simulink model "Core_Model_Cal"  (R2023a)
settings: Solver=FixedStepAuto  StartTime=0  StopTime=Z  FixedStep=1/24  RelTol=1e-3
values from neighbouring files (symbols this model uses):
  c_eh = 0.85    [Model_Parameters.m]
  cc_e = -0.85    [Model_Parameters.m]
  R_H2 = 0.05    [Model_Parameters.m]
  R_lh = 0.025    [Model_Parameters.m]
  R_ng = 0.025    [Model_Parameters.m]
libraries: fl_lib x62, nesl_utility x46, ee_lib x22
settings Model: Creator=pienv  LastModifiedBy=pienv

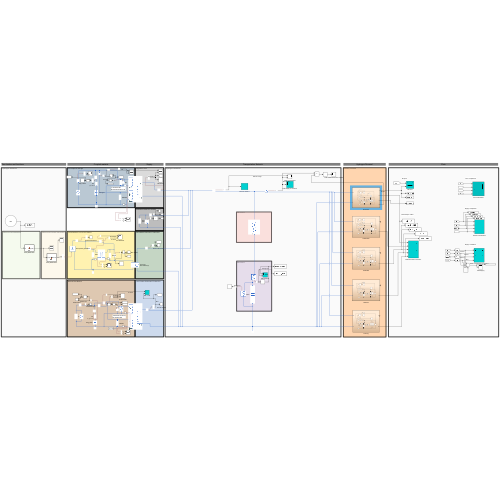
[thumbnail: Simulink's stored preview of the top-level diagram]
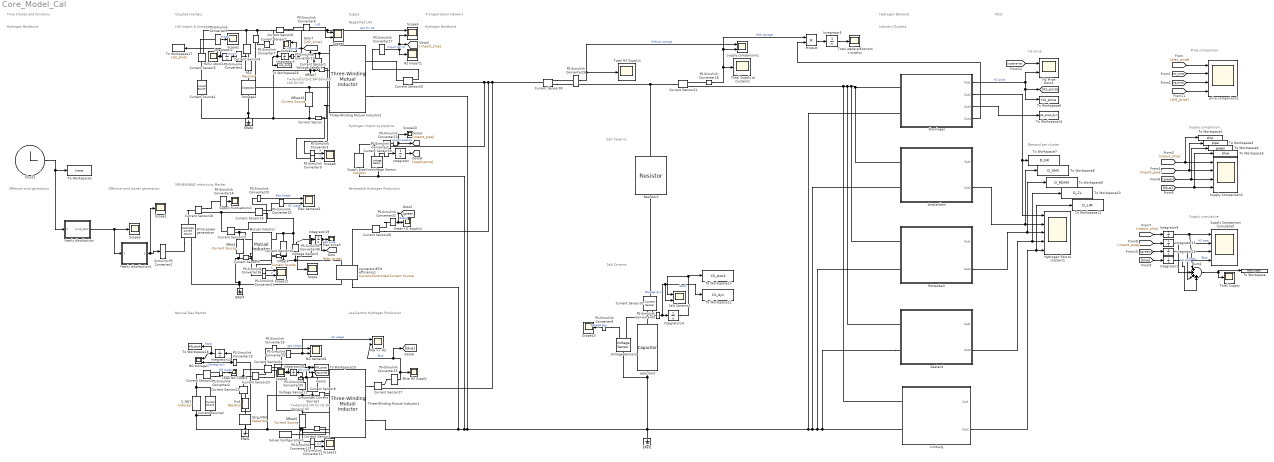
== system Core_Model_Cal ==
  note: Price comparison
  note: Hydrogen Backbone
  note: Supply comparison
  note: Demand per cluster
  note: H2 price
  note: Supply cumulative
  note: Hydrogen Import by pipeline
  note: Renewable Hydrogen Production
  note: Offshore wind generation
  note: Plots
  note: Coupled markets
  note: Natural Gas Market
  note: LH2 Import & storage
  note: Transportation Network
  note: Industry Clusters
  note: Hydrogen Demand
  note: Supply
  note: Offshore wind power generation
  note: Time tracker and functions
  note: T=demand NG for H2
      | B= demand NG
  note: Low-Carbon Hydrogen Production
  note: Salt Caverns
  note: Regasified LH2
  note: Salt Caverns
  note: T=demand LH2
      | B= demand LH2 for H2
  note: Hydrogen Backbone
  note: (RENEWABLE) electricity Market
  Amsterdam : Subsystem
  Blue H2 Supply : Scope
  Clock1 : Clock
      settings: Decimation=24
  Current Sensor{,1..10,17..25,27..28,30..31} (24 alike) : fl_lib/Electrical/Electrical Sensors/Current Sensor
  Current Source1 : ee_lib/Sources/Current Source  dc_current=I_LH2 A  ac_current=0 A  ac_shift=0 rad  ac_frequency=60 Hz  noise_mode=ee.enum.sources.noise.Disabled  PSD=0 A^2/Hz  sample_time=1e-3 s  repeatability=ee.enum.sources.repeatability.NotRepeatable  user_seed=0  auto_seed=3890346746  i_specify=off  i_priority=None  i=0 A  i_nominal_specify=off  i_nominal_unit=A  i_nominal_value=1  v_specify=off  v_priority=None  v=0 V  v_nominal_specify=off  v_nominal_unit=V  v_nominal_value=1
  Current Source2 : ee_lib/Sources/Current Source  dc_current=v_sng A  ac_current=0 A  ac_shift=0 rad  ac_frequency=60 Hz  noise_mode=ee.enum.sources.noise.Disabled  PSD=0 A^2/Hz  sample_time=1e-3 s  repeatability=ee.enum.sources.repeatability.NotRepeatable  user_seed=0  auto_seed=545404223  i_specify=off  i_priority=None  i=0 A  i_nominal_specify=off  i_nominal_unit=A  i_nominal_value=1  v_specify=off  v_priority=None  v=0 V  v_nominal_specify=off  v_nominal_unit=V  v_nominal_value=1
  ERef{1..4} (4 alike) : fl_lib/Electrical/Electrical Elements/Electrical Reference
  Elec demand1 : Scope  NumInputPorts=2
  Elec price3 : Scope
  Green H2 supply1 : Scope
  Groningen : Subsystem
  H2 Import1 : Scope
  H2 Price : Scope  NumInputPorts=2
  H2(L) stock1 : Scope
  Hydrogen flow to clusters1 : Scope  NumInputPorts=5
  Integrator{,1..3,5,9,12,14..16,19..20} (12 alike) : Integrator
  Limburg : Subsystem
  Mutual Inductor : fl_lib/Electrical/Electrical Elements/Mutual Inductor  L1=L_eh H  L2=L_e H  k=cc_e  i1_specify=off  i1_priority=High  i1=0 A  i1_nominal_specify=off  i1_nominal_unit=A  i1_nominal_value=1  i2_specify=off  i2_priority=High  i2=0 A  i2_nominal_specify=off  i2_nominal_unit=A  i2_nominal_value=1  v1_specify=off  v1_priority=None  v1=0 V  v1_nominal_specify=off  v1_nominal_unit=V  v1_nominal_value=1  v2_specify=off  v2_priority=None  v2=0 V  v2_nominal_specify=off  v2_nominal_unit=V  v2_nominal_value=1
      settings: InternalSimscapePortConfiguration="{\"Bottom\":[],\"Left\":[{\"id\":\"p1\",\"label\":\"1+\",\"type\":\"foundation.electrical.electrical\"},{\"id\":\"n1\",\"label\":\"1-\",\"type\":\"foundation.electrical.electrical\"}],\"Right\":[{\"id\":\"p2\",\"label\":\"2+\",\"type\":\"foundation.electrical.electrical\"},{\"id\":\"n2\",\"label\":\"2-\",\"type\":\"foundation.electrical.electrical\"}],\"Top\":[]}"
  NG --> H2 : Scope  NumInputPorts=2
  NG demand1 : Scope  NumInputPorts=2
  NG storage1 : Scope  NumInputPorts=2
  Offset10 : ee_lib/Sources/Current Source  dc_current=id_lh2h A  ac_current=0 A  ac_shift=0 rad  ac_frequency=0 Hz  noise_mode=0  PSD=0 A^2/Hz  sample_time=1e-3 s  repeatability=1  user_seed=0  auto_seed=418932850  i_specify=off  i_priority=None  i=0 A  i_nominal_specify=off  i_nominal_unit=A  i_nominal_value=1  v_specify=off  v_priority=None  v=0 V  v_nominal_specify=off  v_nominal_unit=V  v_nominal_value=1
  Offset4 : ee_lib/Sources/Current Source  dc_current=id_eh A  ac_current=0 A  ac_shift=0 rad  ac_frequency=0 Hz  noise_mode=0  PSD=0 A^2/Hz  sample_time=1e-3 s  repeatability=1  user_seed=0  auto_seed=1196140742  i_specify=off  i_priority=None  i=0 A  i_nominal_specify=off  i_nominal_unit=A  i_nominal_value=1  v_specify=off  v_priority=None  v=0 V  v_nominal_specify=off  v_nominal_unit=V  v_nominal_value=1
  Offset5 : ee_lib/Sources/Current Source  dc_current=id_ngh A  ac_current=0 A  ac_shift=0 rad  ac_frequency=0 Hz  noise_mode=0  PSD=0 A^2/Hz  sample_time=1e-3 s  repeatability=1  user_seed=0  auto_seed=2348838240  i_specify=off  i_priority=None  i=0 A  i_nominal_specify=off  i_nominal_unit=A  i_nominal_value=1  v_specify=off  v_priority=None  v=0 V  v_nominal_specify=off  v_nominal_unit=V  v_nominal_value=1
  Offset7 : ee_lib/Sources/Current Source  dc_current=id_lh2 A  ac_current=0 A  ac_shift=0 rad  ac_frequency=0 Hz  noise_mode=0  PSD=0 A^2/Hz  sample_time=1e-3 s  repeatability=1  user_seed=0  auto_seed=4112460543  i_specify=off  i_priority=None  i=0 A  i_nominal_specify=off  i_nominal_unit=A  i_nominal_value=1  v_specify=off  v_priority=None  v=0 V  v_nominal_specify=off  v_nominal_unit=V  v_nominal_value=1
  Offst3 : ee_lib/Sources/Current Source  dc_current=id_e A  ac_current=0 A  ac_shift=0 rad  ac_frequency=0 Hz  noise_mode=0  PSD=0 A^2/Hz  sample_time=1e-3 s  repeatability=1  user_seed=0  auto_seed=4144164703  i_specify=off  i_priority=None  i=0 A  i_nominal_specify=off  i_nominal_unit=A  i_nominal_value=1  v_specify=off  v_priority=None  v=0 V  v_nominal_specify=off  v_nominal_unit=V  v_nominal_value=1
  PS-Simulink Converter{1..5,8..21,23,25..26,30..33,36} (27 alike) : nesl_utility/PS-Simulink Converter  PhysicalDomain=network_engine_domain  SubClassName=ps_output  LeftPortType=input  RightPortType=output  PseudoPeriodic=off  Frequencies=[]  VectorFormat=1-D array  Unit=1  AffineConversion=off
  PS-Simulink Converter6 : nesl_utility/PS-Simulink Converter  PhysicalDomain=network_engine_domain  SubClassName=ps_output  LeftPortType=input  RightPortType=output  PseudoPeriodic=off  Frequencies=[]  VectorFormat=inherit  Unit=inherit  AffineConversion=off
  PS-Simulink Converter7 : nesl_utility/PS-Simulink Converter  PhysicalDomain=network_engine_domain  SubClassName=ps_output  LeftPortType=input  RightPortType=output  PseudoPeriodic=off  Frequencies=[]  VectorFormat=inherit  Unit=inherit  AffineConversion=off
  Product : Product
  Resistor2 : fl_lib/Electrical/Electrical Elements/Resistor  R=R_H2 Ohm  i_specify=off  i_priority=None  i=0 A  i_nominal_specify=off  i_nominal_unit=A  i_nominal_value=1  v_specify=off  v_priority=None  v=0 V  v_nominal_specify=off  v_nominal_unit=V  v_nominal_value=1
  Rotterdam : Subsystem
  S_NG1 : ee_lib/Passive/Inductor  l=L_sng H  enable_L_tol=ee.enum.toleranceApplication.none  L_tol=20  tol_distribution=ee.enum.toleranceDistribution.uniform  nSigma=4  r=0 Ohm  g=0 1/Ohm  enable_operating_limits=ee.enum.enable.no  operating_limit_action=ee.enum.passive.reportOpLim.warn  max_working_current=1 A  power_rating=1 W  enable_faults=ee.enum.enable.no  fault_action=simscape.enum.assert.action.none  lambdaPercent=50  k_faulted=0.9999  turnsShort=ee.enum.passive.inductor.turnsShortOption.no  openCct=ee.enum.enable.no  groundShort=ee.enum.passive.inductor.groundShortOption.no  groundShortG=0 1/Ohm  tau_fault=1e-3 s  fault_trigger=ee.enum.faults.faultTrigger.temporal  t_fault=1 s  max_permissible_voltage=100 V  n_fail_on_voltage=1  max_permissible_current=1 A  t_fail_on_current=1 s  i_L_specify=off  i_L_priority=High  i_L=0 A  i_L_nominal_specify=off  i_L_nominal_unit=A  i_L_nominal_value=1
  Salt Caverns1 : Scope  NumInputPorts=2
  Scope{,1..3,9..10,13} (7 alike) : Scope
  Scope{4..6,8,11..12} (6 alike) : Scope  NumInputPorts=2
  Simulink-PS Converter2 : nesl_utility/Simulink-PS Converter  PhysicalDomain=network_engine_domain  SubClassName=ps_input  LeftPortType=input  RightPortType=output  PseudoPeriodic=off  Frequencies=[]  NoiseDistribution=none  NoiseParameters=[]  Unit=1  AffineConversion=off  FilteringAndDerivatives=filter  SimscapeFilterOrder=2  InputFilterTimeConstant=0.001  UdotUserProvided=0
  Sinusoidal Current Source1 : ee_lib/Additional Components/SPICE Sources/Sinusoidal Current Source  IO=id_ng_IO A  IA=id_ng_IA A  FREQ=id_ng_FREQ Hz  TD=id_ng_TD s  DF=0 1/s  Gmin_param=ee.enum.gminParam.yes
      settings: InternalSimscapePortConfiguration="{\"Bottom\":[],\"Left\":[{\"id\":\"p\",\"label\":\"+\",\"type\":\"foundation.electrical.electrical\"}],\"Right\":[{\"id\":\"n\",\"label\":\"-\",\"type\":\"foundation.electrical.electrical\"}],\"Top\":[]}"
  Solver Configuration1 : nesl_utility/Solver Configuration  PhysicalDomain=network_engine_domain  SubClassName=solver  LeftPortType=input  RightPortType=generic  Tones=[]  Harmonics=[]  SimulateNoise=off  Profile=off  UseLocalSampling=off  EnableSwitchedLinearOptims=on  FrequencyDomain=off  UseCCode=off  RelTol=0.001  AbsTol=0.001  MinStep=1e-09  ToWorkspace=off  RevertToSquareIcSolve=off  NumHomotopyIterations=100  PhasorMode=off  PhasorModeNumHarmonics=1  ConsistencySolver=NEWTON_XTOL_AFTER_FTOL  IndexReductionMethod=DerivativeReplacement  DoDC=off  ResidualTolerance=1e-09  ConsistencyTolSource=LOCAL  ConsistencyAbsTol=0.001  ConsistencyRelTol=0.001  ConsistencyTolFactor=0.001  UseLocalSolver=off  LocalSolverChoice=NE_BACKWARD_EULER_ADVANCER  ResolveIndetEquations=on  FunctionEvalNumThread=1  LocalSolverSampleTime=0.001  DoFixedCost=off  MaxNonlinIter=3  MaxModeIter=2  ComputeImpulses=off  ImpulseIterations=2  LinearAlgebra=auto  LinearAlgebraNumThread=0  EquationFormulation=NE_TIME_EF  DelaysMemoryBudget=1024  AutomaticFiltering=off  FilteringTimeConstant=0.0001  PartitionStorageMethod=AS_NEEDED  PartitionMemoryBudget=1024  PartitionMethod=ROBUST
  Storage2 : fl_lib/Electrical/Electrical Elements/Capacitor  c=C_lh F  r=0 Ohm  g=0 1/Ohm  i_specify=off  i_priority=None  i=0 A  i_nominal_specify=off  i_nominal_unit=A  i_nominal_value=1  v_specify=off  v_priority=None  v=0 V  v_nominal_specify=off  v_nominal_unit=V  v_nominal_value=1  vc_specify=off  vc_priority=High  vc=0 V  vc_nominal_specify=off  vc_nominal_unit=V  vc_nominal_value=1
  Strg_NG3 : fl_lib/Electrical/Electrical Elements/Capacitor  c=C_ng F  r=0 Ohm  g=0 1/Ohm  i_specify=off  i_priority=None  i=0 A  i_nominal_specify=off  i_nominal_unit=A  i_nominal_value=1  v_specify=off  v_priority=None  v=0 V  v_nominal_specify=off  v_nominal_unit=V  v_nominal_value=1  vc_specify=off  vc_priority=High  vc=0 V  vc_nominal_specify=off  vc_nominal_unit=V  vc_nominal_value=100
  Sum1 : Sum  Inputs=|++++
  Supply pipeline : ee_lib/Passive/Inductor  l=L_i H  enable_L_tol=ee.enum.toleranceApplication.none  L_tol=20  tol_distribution=ee.enum.toleranceDistribution.uniform  nSigma=4  r=0 Ohm  g=0 1/Ohm  enable_operating_limits=ee.enum.enable.no  operating_limit_action=ee.enum.passive.reportOpLim.warn  max_working_current=1 A  power_rating=1 W  enable_faults=ee.enum.enable.no  fault_action=simscape.enum.assert.action.none  lambdaPercent=50  k_faulted=0.9999  turnsShort=ee.enum.passive.inductor.turnsShortOption.no  openCct=ee.enum.enable.no  groundShort=ee.enum.passive.inductor.groundShortOption.no  groundShortG=0 1/Ohm  tau_fault=1e-3 s  fault_trigger=ee.enum.faults.faultTrigger.temporal  t_fault=1 s  max_permissible_voltage=100 V  n_fail_on_voltage=1  max_permissible_current=1 A  t_fail_on_current=1 s  i_L_specify=off  i_L_priority=High  i_L=0 A  i_L_nominal_specify=off  i_L_nominal_unit=A  i_L_nominal_value=1
  Supply Comparison Cumulatief : Scope  NumInputPorts=4
  Supply Comparison3 : Scope  NumInputPorts=4
  Supply fluctuations1 : Scope
  Three-Winding Mutual Inductor1 : ee_lib/Passive/Transformers/Three-Winding Mutual Inductor  L1=L_sbh H  L2=L_ngh H  L3=L_ng H  K12=c_ng12  K13=c_ng13  K23=c_ng23  IC_given=1  IC1=0 A  IC2=0 A  IC3=0 A
      settings: LogSimulationData=on  InternalSimscapePortConfiguration="{\"Bottom\":[],\"Left\":[{\"id\":\"p1\",\"label\":\"1+\",\"type\":\"foundation.electrical.electrical\"},{\"id\":\"n1\",\"label\":\"1-\",\"type\":\"foundation.electrical.electrical\"}],\"Right\":[{\"id\":\"p2\",\"label\":\"2+\",\"type\":\"foundation.electrical.electrical\"},{\"id\":\"n2\",\"label\":\"2-\",\"type\":\"foundation.electrical.electrical\"},{\"id\":\"p3\",\"label\":\"3+\",\"type\":\"foundation.electrical.electrical\"},{\"id\":\"n3\",\"label\":\"3-\",\"type\":\"foundation.electrical.electrical\"}],\"Top\":[]}"
  Three-Winding Mutual Inductor2 : ee_lib/Passive/Transformers/Three-Winding Mutual Inductor  L1=L_sih H  L2=L_lh2h H  L3=L_lh2 H  K12=c_lh212  K13=c_lh213  K23=c_lh223  IC_given=1  IC1=0 A  IC2=0 A  IC3=0 A
      settings: LogSimulationData=on  InternalSimscapePortConfiguration="{\"Bottom\":[],\"Left\":[{\"id\":\"p1\",\"label\":\"1+\",\"type\":\"foundation.electrical.electrical\"},{\"id\":\"n1\",\"label\":\"1-\",\"type\":\"foundation.electrical.electrical\"}],\"Right\":[{\"id\":\"p2\",\"label\":\"2+\",\"type\":\"foundation.electrical.electrical\"},{\"id\":\"n2\",\"label\":\"2-\",\"type\":\"foundation.electrical.electrical\"},{\"id\":\"p3\",\"label\":\"3+\",\"type\":\"foundation.electrical.electrical\"},{\"id\":\"n3\",\"label\":\"3-\",\"type\":\"foundation.electrical.electrical\"}],\"Top\":[]}"
  To Workspace : ToWorkspace  VariableName=total_supply  SampleTime=-1
  To Workspace1 : ToWorkspace  VariableName=time  SampleTime=-1
  To Workspace10 : ToWorkspace  VariableName=D_ZL  SampleTime=-1
      settings: Save2DSignal=2-D array (concatenate along first dimension)
  To Workspace11 : ToWorkspace  VariableName=D_LIM  SampleTime=-1
      settings: Save2DSignal=2-D array (concatenate along first dimension)
  To Workspace12 : ToWorkspace  VariableName=CS_dyn  SampleTime=-1
      settings: Save2DSignal=2-D array (concatenate along first dimension)
  To Workspace13 : ToWorkspace  VariableName=CS_stock  SampleTime=-1
  To Workspace14 : ToWorkspace  VariableName=H2_price_dyn  SampleTime=-1
      settings: Save2DSignal=2-D array (concatenate along first dimension)
  To Workspace15 : ToWorkspace  VariableName=NG_price  SampleTime=-1
      settings: Save2DSignal=2-D array (concatenate along first dimension)
  To Workspace16 : ToWorkspace  VariableName=LH2_price  SampleTime=-1
  To Workspace17 : ToWorkspace  VariableName=LH2_stock  SampleTime=-1
  To Workspace18 : ToWorkspace  VariableName=NG_stock  SampleTime=-1
  To Workspace2 : ToWorkspace  VariableName=ship  SampleTime=-1
  To Workspace3 : ToWorkspace  VariableName=pipe  SampleTime=-1
  To Workspace4 : ToWorkspace  VariableName=green  SampleTime=-1
  To Workspace5 : ToWorkspace  VariableName=blue  SampleTime=-1
  To Workspace6 : ToWorkspace  VariableName=H2_price  SampleTime=-1
  To Workspace7 : ToWorkspace  VariableName=D_GR  SampleTime=-1
      settings: Save2DSignal=2-D array (concatenate along first dimension)
  To Workspace8 : ToWorkspace  VariableName=D_AMS  SampleTime=-1
      settings: Save2DSignal=2-D array (concatenate along first dimension)
  To Workspace9 : ToWorkspace  VariableName=D_RDAM  SampleTime=-1
      settings: Save2DSignal=2-D array (concatenate along first dimension)
  Total H2 Supply1 : Scope
  Total NG Supply : Scope
  Total Supply : Scope
  Total Supply to clusters1 : Scope
  Total welfare/Economic surplus : Scope
  Voltage Sensor{,1..2,5,11} (5 alike) : fl_lib/Electrical/Electrical Sensors/Voltage Sensor
  Wind power generation : fl_lib/Electrical/Electrical Sources/Controlled Current Source
  Yearly distribution : MATLAB Function  TreatAsAtomicUnit=on
  Yearly distribution1 : MATLAB Function  TreatAsAtomicUnit=on
  Zeeland : Subsystem
  apacitor2 : fl_lib/Electrical/Electrical Elements/Capacitor  c=C_sc F  r=0 Ohm  g=0 1/Ohm  i_specify=on  i_priority=None  i=0.1 A  i_nominal_specify=off  i_nominal_unit=A  i_nominal_value=0.1  v_specify=off  v_priority=None  v=0 V  v_nominal_specify=off  v_nominal_unit=V  v_nominal_value=1  vc_specify=off  vc_priority=High  vc=0 V  vc_nominal_specify=off  vc_nominal_unit=V  vc_nominal_value=1
  conversie 85% efficiency1 : fl_lib/Electrical/Electrical Sources/Current-Controlled Current Source  K=c_eh  i1_specify=off  i1_priority=None  i1=0 A  i1_nominal_specify=off  i1_nominal_unit=A  i1_nominal_value=1  i2_specify=off  i2_priority=None  i2=0 A  i2_nominal_specify=off  i2_nominal_unit=A  i2_nominal_value=1
      settings: InternalSimscapePortConfiguration="{\"Bottom\":[],\"Left\":[{\"id\":\"p1\",\"label\":\"+\",\"type\":\"foundation.electrical.electrical\"},{\"id\":\"head\",\"label\":\"\",\"type\":\"foundation.electrical.electrical\"}],\"Right\":[{\"id\":\"n1\",\"label\":\"-\",\"type\":\"foundation.electrical.electrical\"},{\"id\":\"tail\",\"label\":\"\",\"type\":\"foundation.electrical.electrical\"}],\"Top\":[]}"
  frc2 : fl_lib/Electrical/Electrical Elements/Resistor  R=R_lh Ohm  i_specify=off  i_priority=High  i=0 A  i_nominal_specify=off  i_nominal_unit=A  i_nominal_value=1  v_specify=off  v_priority=High  v=0 V  v_nominal_specify=off  v_nominal_unit=V  v_nominal_value=1
      settings: AttributesFormatString=%<R> %<R_unit>
  frc4 : fl_lib/Electrical/Electrical Elements/Resistor  R=R_ng Ohm  i_specify=off  i_priority=High  i=0 A  i_nominal_specify=off  i_nominal_unit=A  i_nominal_value=1  v_specify=off  v_priority=High  v=0 V  v_nominal_specify=off  v_nominal_unit=V  v_nominal_value=1
      settings: AttributesFormatString=%<R> %<R_unit>
  price comparison1 : Scope  NumInputPorts=4
  supply comparison1 : Scope  NumInputPorts=2
  wires:
  Integrator2/1 -> To Workspace17/1, H2(L) stock1/1
  Clock1/1 -> Yearly distribution/1(X), To Workspace1/1
  [LH2_price] -> price comparison1/4
  Integrator3/1 -> To Workspace16/1, Scope6/1, [LH2_price]  "LH2 price"
  PS-Simulink Converter10/1 -> Integrator3/1
  [import_pipe] -> To Workspace3/1, Supply Comparison3/2
  [green] -> To Workspace4/1, Supply Comparison3/3
  Integrator14/1 -> To Workspace13/1, Salt Caverns1/1  "Stock"
  Yearly distribution1/1(current) -> Scope1/1, Simulink-PS Converter2/1
  PS-Simulink Converter19/1 -> Integrator12/1, NG storage1/2  "Storage dyn"
  Groningen/2(Out2) -> Hydrogen flow to clusters1/1, To Workspace7/1
  PS-Simulink Converter32/1 -> Elec demand1/2  "H2 usage"
  Limburg/2(Out2) -> To Workspace11/1, Hydrogen flow to clusters1/5
  Zeeland/2(Out2) -> Hydrogen flow to clusters1/4, To Workspace10/1
  PS-Simulink Converter25/1 -> NG demand1/1  "gas Usage"
  PS-Simulink Converter23/1 -> NG --> H2/1, NG demand1/2  "H2 usage"
  PS-Simulink Converter31/1 -> [green], Green H2 supply1/1  "Green"
  Amsterdam/2(Out2) -> To Workspace8/1, Hydrogen flow to clusters1/2
  PS-Simulink Converter36/1 -> Scope/1, Integrator19/1
  PS-Simulink Converter20/1 -> Elec demand1/1  "Elec Usage"
  Rotterdam/2(Out2) -> Hydrogen flow to clusters1/3, To Workspace9/1
  PS-Simulink Converter30/1 -> Integrator20/1
  PS-Simulink Converter2/1 -> Total NG Supply/1  "NG supply"
  PS-Simulink Converter15/1 -> [blue], NG --> H2/2, Blue H2 Supply/1  "Blue"
  PS-Simulink Converter13/1 -> Scope10/1, [import_pipe]  "import pipeline"
  Groningen/3(Out3) -> To Workspace14/1
  Integrator/1 -> [supplyprice]
  PS-Simulink Converter14/1 -> Supply fluctuations1/1
  Integrator19/1 -> [elec_price], Elec price3/1  "elec price"
  Integrator15/1 -> Supply Comparison Cumulatief/2, Sum1/2  "H2 pipe"
  PS-Simulink Converter6/1 -> Scope4/2  "LH2"
  [supplyprice] -> H2 Price/1
  [import_ship] -> Integrator9/1
  PS-Simulink Converter26/1 -> supply comparison1/1, Total H2 Supply1/1  "Without storage"
  Integrator12/1 -> To Workspace18/1, NG storage1/1  "Stock"
  [blue] -> Integrator1/1
  Integrator16/1 -> Supply Comparison Cumulatief/3, Sum1/3  "Green"
  [blue] -> To Workspace5/1, Supply Comparison3/4
  [import_pipe] -> Integrator15/1
  [import_ship] -> To Workspace2/1, Supply Comparison3/1
  Sum1/1 -> Total Supply/1, To Workspace/1
  [ng_price] -> price comparison1/3
  PS-Simulink Converter4/1 -> Integrator2/1  "Import"
  PS-Simulink Converter17/1 -> Scope5/2, [import_ship], H2 Import1/1  "Import H2 (L)"
  Integrator1/1 -> Supply Comparison Cumulatief/4, Sum1/4  "Blue"
  PS-Simulink Converter7/1 -> Scope5/1, Scope4/1  "LH2 for H2"
  Groningen/1(Out1) -> H2 Price/2, To Workspace6/1, [H2_price]  "H2 price"
  Integrator9/1 -> Supply Comparison Cumulatief/1, Sum1/1  "H2 ship"
  PS-Simulink Converter33/1 -> To Workspace12/1, Salt Caverns1/2, Integrator14/1  "Storage dyn"
  [green] -> Integrator16/1
  [H2_price] -> price comparison1/2
  PS-Simulink Converter18/1 -> Product/1, supply comparison1/2, Total Supply to clusters1/1  "With storage"
  PS-Simulink Converter5/1 -> Scope2/1  "Import"
  [elec_price] -> price comparison1/1
  Integrator20/1 -> [ng_price], To Workspace15/1, Scope9/1  "NG price"
  PS-Simulink Converter1/1 -> Integrator/1
  Yearly distribution/1(wind_distr) -> Yearly distribution1/1(wind_distr), Scope3/1
  PS-Simulink Converter3/1 -> Scope8/1  "3"
  PS-Simulink Converter9/1 -> Scope8/2  "2"
  PS-Simulink Converter11/1 -> Scope11/1  "3"
  PS-Simulink Converter12/1 -> Scope11/2  "2"
  PS-Simulink Converter16/1 -> Scope12/1  "1"
  PS-Simulink Converter21/1 -> Scope12/2  "2"
  Groningen/4(Out4) -> Product/2
  Product/1 -> Integrator5/1
  Integrator5/1 -> Total welfare/Economic surplus/1
  PS-Simulink Converter8/1 -> Scope13/1  "Storage dyn"
  connections:
  ERef4/LConn1 -- Current Sensor/LConn1 -- Offset10/LConn1 -- Voltage Sensor1/LConn1 -- Current Sensor1/LConn1 -- Offset7/LConn1 -- Current Source1/RConn1 -- Storage2/LConn1
  Voltage Sensor5/RConn2 -- Current Sensor25/RConn2 -- Mutual Inductor/LConn2 -- Offset4/RConn1
  Current Sensor28/RConn2 -- Current Sensor30/LConn1 -- Current Sensor17/RConn2 -- Current Sensor20/RConn2 -- Current Sensor19/RConn2
  Voltage Sensor11/RConn2 -- Current Sensor23/RConn2 -- Sinusoidal Current Source1/LConn1 -- Three-Winding Mutual Inductor1/RConn4
  Offset5/LConn1 -- Current Sensor3/LConn1 -- Current Source2/RConn1 -- S_NG1/LConn1 -- Strg_NG3/LConn1 -- ERef2/LConn1 -- Sinusoidal Current Source1/RConn1 -- Current Sensor8/LConn1 -- Voltage Sensor11/LConn1 -- Solver Configuration1/RConn1
  Current Sensor24/RConn2 -- Three-Winding Mutual Inductor1/RConn2 -- Offset5/RConn1
  Voltage Sensor5/LConn1 -- Offset4/LConn1 -- Current Sensor10/LConn1 -- conversie 85% efficiency1/LConn1
  Limburg/LConn1 -- Current Sensor21/RConn2 -- Amsterdam/LConn1 -- Groningen/LConn1 -- Rotterdam/LConn1 -- Zeeland/LConn1
  Zeeland/LConn2 -- Limburg/LConn2 -- Voltage Sensor2/LConn1 -- apacitor2/LConn1 -- Supply pipeline/LConn1 -- Voltage Sensor/LConn1 -- conversie 85% efficiency1/RConn2 -- Three-Winding Mutual Inductor1/LConn1 -- Three-Winding Mutual Inductor2/LConn1 -- ERef1/LConn1 -- Groningen/LConn2 -- Amsterdam/LConn2 -- Rotterdam/LConn2
  Current Sensor21/LConn1 -- Resistor2/RConn1 -- Current Sensor30/RConn2
  Current Sensor22/LConn1 -- Current Sensor2/RConn2 -- Current Sensor24/LConn1 -- Current Sensor23/LConn1
  Current Sensor6/LConn1 -- Current Sensor7/LConn1 -- Current Sensor4/LConn1 -- Current Sensor5/RConn2
  Offset7/RConn1 -- Current Sensor6/RConn2 -- Three-Winding Mutual Inductor2/RConn4 -- Voltage Sensor1/RConn2
  Wind power generation/RConn2 -- conversie 85% efficiency1/RConn1 -- Offst3/LConn1 -- Current Sensor9/LConn1 -- ERef3/LConn1
  Current Sensor25/LConn1 -- Current Sensor27/LConn1 -- Current Sensor18/RConn2
  Current Sensor2/LConn1 -- S_NG1/RConn1 -- Current Source2/LConn1
  Current Sensor19/LConn1 -- Supply pipeline/RConn1 -- Voltage Sensor/RConn2
  Current Sensor5/LConn1 -- Current Source1/LConn1
  Current Sensor27/RConn2 -- Mutual Inductor/RConn2 -- Offst3/RConn1
  Offset10/RConn1 -- Current Sensor7/RConn2 -- Three-Winding Mutual Inductor2/RConn2
  PS-Simulink Converter4/LConn1 -- Current Sensor4/RConn1
  frc2/RConn1 -- Current Sensor4/RConn2
  PS-Simulink Converter2/LConn1 -- Current Sensor2/RConn1
  PS-Simulink Converter23/LConn1 -- Current Sensor24/RConn1
  Current Sensor22/RConn2 -- frc4/RConn1
  Current Sensor28/LConn1 -- conversie 85% efficiency1/LConn2
  PS-Simulink Converter31/LConn1 -- Current Sensor28/RConn1
  Current Sensor31/RConn2 -- Voltage Sensor2/RConn2 -- apacitor2/RConn1
  PS-Simulink Converter33/LConn1 -- Current Sensor31/RConn1
  frc4/LConn1 -- Strg_NG3/RConn1
  PS-Simulink Converter10/LConn1 -- Voltage Sensor1/RConn1
  Current Sensor18/RConn1 -- PS-Simulink Converter14/LConn1
  PS-Simulink Converter18/LConn1 -- Current Sensor21/RConn1
  Current Sensor27/RConn1 -- PS-Simulink Converter20/LConn1
  PS-Simulink Converter7/LConn1 -- Current Sensor7/RConn1
  PS-Simulink Converter13/LConn1 -- Current Sensor19/RConn1
  PS-Simulink Converter25/LConn1 -- Current Sensor23/RConn1
  Current Sensor22/RConn1 -- PS-Simulink Converter19/LConn1
  Storage2/RConn1 -- frc2/LConn1
  PS-Simulink Converter1/LConn1 -- Voltage Sensor/RConn1
  PS-Simulink Converter36/LConn1 -- Voltage Sensor5/RConn1
  PS-Simulink Converter6/LConn1 -- Current Sensor6/RConn1
  Three-Winding Mutual Inductor2/LConn2 -- Current Sensor20/LConn1
  PS-Simulink Converter15/LConn1 -- Current Sensor17/RConn1
  PS-Simulink Converter17/LConn1 -- Current Sensor20/RConn1
  Three-Winding Mutual Inductor1/LConn2 -- Current Sensor17/LConn1
  PS-Simulink Converter30/LConn1 -- Voltage Sensor11/RConn1
  Resistor2/LConn1 -- Current Sensor31/LConn1
  Current Sensor30/RConn1 -- PS-Simulink Converter26/LConn1
  PS-Simulink Converter5/LConn1 -- Current Sensor5/RConn1
  PS-Simulink Converter32/LConn1 -- Current Sensor25/RConn1
  Current Sensor18/LConn1 -- Wind power generation/LConn1
  Three-Winding Mutual Inductor2/RConn1 -- Current Sensor/RConn2
  Current Sensor1/RConn2 -- Three-Winding Mutual Inductor2/RConn3
  PS-Simulink Converter3/LConn1 -- Current Sensor1/RConn1
  PS-Simulink Converter9/LConn1 -- Current Sensor/RConn1
  PS-Simulink Converter11/LConn1 -- Current Sensor8/RConn1
  PS-Simulink Converter12/LConn1 -- Current Sensor3/RConn1
  Three-Winding Mutual Inductor1/RConn3 -- Current Sensor8/RConn2
  Three-Winding Mutual Inductor1/RConn1 -- Current Sensor3/RConn2
  Current Sensor9/RConn2 -- Mutual Inductor/RConn1
  Current Sensor9/RConn1 -- PS-Simulink Converter21/LConn1
  Current Sensor10/RConn2 -- Mutual Inductor/LConn1
  Current Sensor10/RConn1 -- PS-Simulink Converter16/LConn1
  PS-Simulink Converter8/LConn1 -- Voltage Sensor2/RConn1
  Wind power generation/RConn1 -- Simulink-PS Converter2/RConn1

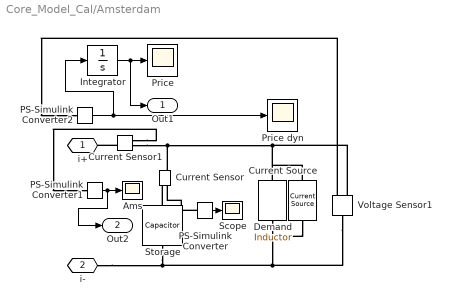
== system Core_Model_Cal/Amsterdam ==
  Ams : Scope
  Current Sensor : fl_lib/Electrical/Electrical Sensors/Current Sensor
  Current Sensor1 : fl_lib/Electrical/Electrical Sensors/Current Sensor
  Current Source : ee_lib/Sources/Current Source  dc_current=id_a A  ac_current=0 A  ac_shift=0 rad  ac_frequency=0 Hz  noise_mode=ee.enum.sources.noise.Disabled  PSD=0 A^2/Hz  sample_time=1e-3 s  repeatability=ee.enum.sources.repeatability.NotRepeatable  user_seed=0  auto_seed=3499211588  i_specify=off  i_priority=None  i=0 A  i_nominal_specify=off  i_nominal_unit=A  i_nominal_value=1  v_specify=off  v_priority=None  v=0 V  v_nominal_specify=off  v_nominal_unit=V  v_nominal_value=1
  Demand : ee_lib/Passive/Inductor  l=L_a H  enable_L_tol=0  L_tol=20  tol_distribution=1  nSigma=4  r=0 Ohm  g=0 1/Ohm  enable_operating_limits=0  operating_limit_action=2  max_working_current=1 A  power_rating=1 W  enable_faults=ee.enum.enable.no  fault_action=simscape.enum.assert.action.none  lambdaPercent=50  k_faulted=0.9999  turnsShort=0  openCct=0  groundShort=0  groundShortG=0 1/Ohm  tau_fault=1e-3 s  fault_trigger=ee.enum.faults.faultTrigger.temporal  t_fault=1 s  max_permissible_voltage=100 V  n_fail_on_voltage=1  max_permissible_current=1 A  t_fail_on_current=1 s  i_L_specify=off  i_L_priority=High  i_L=0 A  i_L_nominal_specify=off  i_L_nominal_unit=A  i_L_nominal_value=1
  Integrator : Integrator
  PS-Simulink Converter : nesl_utility/PS-Simulink Converter  PhysicalDomain=network_engine_domain  SubClassName=ps_output  LeftPortType=input  RightPortType=output  PseudoPeriodic=off  Frequencies=[]  VectorFormat=inherit  Unit=inherit  AffineConversion=off
  PS-Simulink Converter1 : nesl_utility/PS-Simulink Converter  PhysicalDomain=network_engine_domain  SubClassName=ps_output  LeftPortType=input  RightPortType=output  PseudoPeriodic=off  Frequencies=[]  VectorFormat=inherit  Unit=inherit  AffineConversion=off
  PS-Simulink Converter2 : nesl_utility/PS-Simulink Converter  PhysicalDomain=network_engine_domain  SubClassName=ps_output  LeftPortType=input  RightPortType=output  PseudoPeriodic=off  Frequencies=[]  VectorFormat=inherit  Unit=inherit  AffineConversion=off
  "Price " : Scope
  Price dyn : Scope
  Scope : Scope
  Storage : fl_lib/Electrical/Electrical Elements/Capacitor  c=C_a F  r=0 Ohm  g=0 1/Ohm  i_specify=off  i_priority=None  i=0 A  i_nominal_specify=off  i_nominal_unit=A  i_nominal_value=1  v_specify=off  v_priority=None  v=0 V  v_nominal_specify=off  v_nominal_unit=V  v_nominal_value=1  vc_specify=off  vc_priority=High  vc=0 V  vc_nominal_specify=off  vc_nominal_unit=V  vc_nominal_value=1
  Voltage Sensor1 : fl_lib/Electrical/Electrical Sensors/Voltage Sensor
  "i+ " : PMIOPort  Tag=PMCPort  Side=Left
  i- : PMIOPort  Tag=PMCPort  Port=2  Side=Left
  Out1 : Outport
  Out2 : Outport  Port=2
  wires:
  Integrator/1 -> Out1/1, "Price "/1
  PS-Simulink Converter/1 -> Scope/1
  PS-Simulink Converter2/1 -> Integrator/1, Price dyn/1
  PS-Simulink Converter1/1 -> Out2/1, Ams/1
  connections:
  Demand/LConn1 -- i-/RConn1 -- Storage/LConn1 -- Voltage Sensor1/LConn1 -- Current Source/LConn1
  Current Sensor/LConn1 -- Voltage Sensor1/RConn2 -- Current Source/RConn1 -- Demand/RConn1 -- Current Sensor1/RConn2
  Storage/RConn1 -- Current Sensor/RConn2
  Voltage Sensor1/RConn1 -- PS-Simulink Converter2/LConn1
  PS-Simulink Converter/LConn1 -- Current Sensor/RConn1
  Current Sensor1/RConn1 -- PS-Simulink Converter1/LConn1
  Current Sensor1/LConn1 -- "i+ "/RConn1

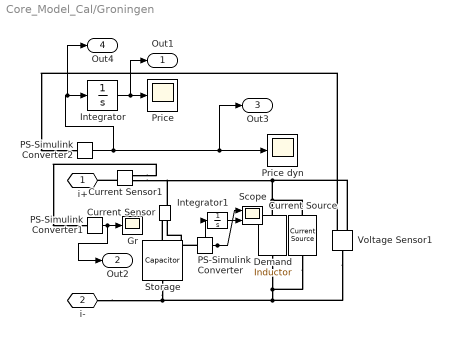
== system Core_Model_Cal/Groningen ==
  Current Sensor : fl_lib/Electrical/Electrical Sensors/Current Sensor
  Current Sensor1 : fl_lib/Electrical/Electrical Sensors/Current Sensor
  Current Source : ee_lib/Sources/Current Source  dc_current=id_g A  ac_current=0 A  ac_shift=0 rad  ac_frequency=0 Hz  noise_mode=ee.enum.sources.noise.Disabled  PSD=0 A^2/Hz  sample_time=1e-3 s  repeatability=ee.enum.sources.repeatability.NotRepeatable  user_seed=0  auto_seed=3922919431  i_specify=off  i_priority=None  i=0 A  i_nominal_specify=off  i_nominal_unit=A  i_nominal_value=1  v_specify=off  v_priority=None  v=0 V  v_nominal_specify=off  v_nominal_unit=V  v_nominal_value=1
  Demand : ee_lib/Passive/Inductor  l=L_g H  enable_L_tol=0  L_tol=20  tol_distribution=1  nSigma=4  r=0 Ohm  g=0 1/Ohm  enable_operating_limits=0  operating_limit_action=2  max_working_current=1 A  power_rating=1 W  enable_faults=ee.enum.enable.no  fault_action=simscape.enum.assert.action.none  lambdaPercent=50  k_faulted=0.9999  turnsShort=0  openCct=0  groundShort=0  groundShortG=0 1/Ohm  tau_fault=1e-3 s  fault_trigger=ee.enum.faults.faultTrigger.temporal  t_fault=1 s  max_permissible_voltage=100 V  n_fail_on_voltage=1  max_permissible_current=1 A  t_fail_on_current=1 s  i_L_specify=off  i_L_priority=High  i_L=0 A  i_L_nominal_specify=off  i_L_nominal_unit=A  i_L_nominal_value=1
  Gr : Scope
  Integrator : Integrator
  Integrator1 : Integrator
  PS-Simulink Converter : nesl_utility/PS-Simulink Converter  PhysicalDomain=network_engine_domain  SubClassName=ps_output  LeftPortType=input  RightPortType=output  PseudoPeriodic=off  Frequencies=[]  VectorFormat=inherit  Unit=inherit  AffineConversion=off
  PS-Simulink Converter1 : nesl_utility/PS-Simulink Converter  PhysicalDomain=network_engine_domain  SubClassName=ps_output  LeftPortType=input  RightPortType=output  PseudoPeriodic=off  Frequencies=[]  VectorFormat=inherit  Unit=inherit  AffineConversion=off
  PS-Simulink Converter2 : nesl_utility/PS-Simulink Converter  PhysicalDomain=network_engine_domain  SubClassName=ps_output  LeftPortType=input  RightPortType=output  PseudoPeriodic=off  Frequencies=[]  VectorFormat=inherit  Unit=inherit  AffineConversion=off
  "Price " : Scope
  Price dyn : Scope
  Scope : Scope  NumInputPorts=2
  Storage : fl_lib/Electrical/Electrical Elements/Capacitor  c=C_g F  r=0 Ohm  g=0 1/Ohm  i_specify=off  i_priority=None  i=0 A  i_nominal_specify=off  i_nominal_unit=A  i_nominal_value=1  v_specify=off  v_priority=None  v=0 V  v_nominal_specify=off  v_nominal_unit=V  v_nominal_value=1  vc_specify=off  vc_priority=High  vc=0 V  vc_nominal_specify=off  vc_nominal_unit=V  vc_nominal_value=1
  Voltage Sensor1 : fl_lib/Electrical/Electrical Sensors/Voltage Sensor
  "i+ " : PMIOPort  Tag=PMCPort  Side=Left
  i- : PMIOPort  Tag=PMCPort  Port=2  Side=Left
  Out1 : Outport
  Out2 : Outport  Port=2
  Out3 : Outport  Port=3
  Out4 : Outport  Port=4
  wires:
  PS-Simulink Converter2/1 -> Out4/1, Integrator/1, Out3/1, Price dyn/1
  Integrator/1 -> Out1/1, "Price "/1
  PS-Simulink Converter1/1 -> Out2/1, Gr/1
  PS-Simulink Converter/1 -> Scope/1, Integrator1/1
  Integrator1/1 -> Scope/2
  connections:
  Demand/LConn1 -- Current Source/LConn1 -- Voltage Sensor1/LConn1 -- i-/RConn1 -- Storage/LConn1
  Demand/RConn1 -- Voltage Sensor1/RConn2 -- Current Sensor1/RConn2 -- Current Sensor/LConn1 -- Current Source/RConn1
  PS-Simulink Converter/LConn1 -- Current Sensor/RConn1
  Storage/RConn1 -- Current Sensor/RConn2
  Voltage Sensor1/RConn1 -- PS-Simulink Converter2/LConn1
  Current Sensor1/LConn1 -- "i+ "/RConn1
  Current Sensor1/RConn1 -- PS-Simulink Converter1/LConn1

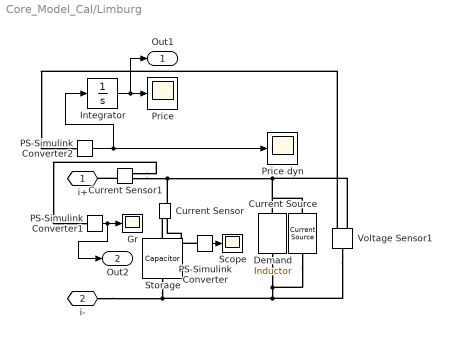
== system Core_Model_Cal/Limburg ==
  Current Sensor : fl_lib/Electrical/Electrical Sensors/Current Sensor
  Current Sensor1 : fl_lib/Electrical/Electrical Sensors/Current Sensor
  Current Source : ee_lib/Sources/Current Source  dc_current=id_l A  ac_current=0 A  ac_shift=0 rad  ac_frequency=0 Hz  noise_mode=ee.enum.sources.noise.Disabled  PSD=0 A^2/Hz  sample_time=1e-3 s  repeatability=ee.enum.sources.repeatability.NotRepeatable  user_seed=0  auto_seed=2715962282  i_specify=off  i_priority=None  i=0 A  i_nominal_specify=off  i_nominal_unit=A  i_nominal_value=1  v_specify=off  v_priority=None  v=0 V  v_nominal_specify=off  v_nominal_unit=V  v_nominal_value=1
  Demand : ee_lib/Passive/Inductor  l=L_l H  enable_L_tol=0  L_tol=20  tol_distribution=1  nSigma=4  r=0 Ohm  g=0 1/Ohm  enable_operating_limits=0  operating_limit_action=2  max_working_current=1 A  power_rating=1 W  enable_faults=ee.enum.enable.no  fault_action=simscape.enum.assert.action.none  lambdaPercent=50  k_faulted=0.9999  turnsShort=0  openCct=0  groundShort=0  groundShortG=0 1/Ohm  tau_fault=1e-3 s  fault_trigger=ee.enum.faults.faultTrigger.temporal  t_fault=1 s  max_permissible_voltage=100 V  n_fail_on_voltage=1  max_permissible_current=1 A  t_fail_on_current=1 s  i_L_specify=off  i_L_priority=High  i_L=0 A  i_L_nominal_specify=off  i_L_nominal_unit=A  i_L_nominal_value=1
  Gr : Scope
  Integrator : Integrator
  PS-Simulink Converter : nesl_utility/PS-Simulink Converter  PhysicalDomain=network_engine_domain  SubClassName=ps_output  LeftPortType=input  RightPortType=output  PseudoPeriodic=off  Frequencies=[]  VectorFormat=inherit  Unit=inherit  AffineConversion=off
  PS-Simulink Converter1 : nesl_utility/PS-Simulink Converter  PhysicalDomain=network_engine_domain  SubClassName=ps_output  LeftPortType=input  RightPortType=output  PseudoPeriodic=off  Frequencies=[]  VectorFormat=inherit  Unit=inherit  AffineConversion=off
  PS-Simulink Converter2 : nesl_utility/PS-Simulink Converter  PhysicalDomain=network_engine_domain  SubClassName=ps_output  LeftPortType=input  RightPortType=output  PseudoPeriodic=off  Frequencies=[]  VectorFormat=inherit  Unit=inherit  AffineConversion=off
  "Price " : Scope
  Price dyn : Scope
  Scope : Scope
  Storage : fl_lib/Electrical/Electrical Elements/Capacitor  c=C_l F  r=0 Ohm  g=0 1/Ohm  i_specify=off  i_priority=None  i=0 A  i_nominal_specify=off  i_nominal_unit=A  i_nominal_value=1  v_specify=off  v_priority=None  v=0 V  v_nominal_specify=off  v_nominal_unit=V  v_nominal_value=1  vc_specify=off  vc_priority=High  vc=0 V  vc_nominal_specify=off  vc_nominal_unit=V  vc_nominal_value=1
  Voltage Sensor1 : fl_lib/Electrical/Electrical Sensors/Voltage Sensor
  "i+ " : PMIOPort  Tag=PMCPort  Side=Left
  i- : PMIOPort  Tag=PMCPort  Port=2  Side=Left
  Out1 : Outport
  Out2 : Outport  Port=2
  wires:
  Integrator/1 -> Out1/1, "Price "/1
  PS-Simulink Converter/1 -> Scope/1
  PS-Simulink Converter2/1 -> Integrator/1, Price dyn/1
  PS-Simulink Converter1/1 -> Out2/1, Gr/1
  connections:
  Demand/LConn1 -- Current Source/LConn1 -- i-/RConn1 -- Storage/LConn1 -- Voltage Sensor1/LConn1
  Current Sensor/LConn1 -- Voltage Sensor1/RConn2 -- Current Source/RConn1 -- Demand/RConn1 -- Current Sensor1/RConn2
  Storage/RConn1 -- Current Sensor/RConn2
  Voltage Sensor1/RConn1 -- PS-Simulink Converter2/LConn1
  PS-Simulink Converter/LConn1 -- Current Sensor/RConn1
  Current Sensor1/RConn1 -- PS-Simulink Converter1/LConn1
  Current Sensor1/LConn1 -- "i+ "/RConn1

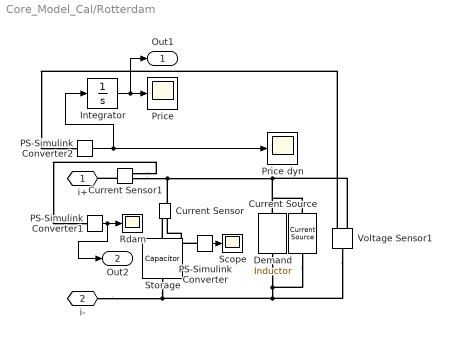
== system Core_Model_Cal/Rotterdam ==
  Current Sensor : fl_lib/Electrical/Electrical Sensors/Current Sensor
  Current Sensor1 : fl_lib/Electrical/Electrical Sensors/Current Sensor
  Current Source : ee_lib/Sources/Current Source  dc_current=id_r A  ac_current=0 A  ac_shift=0 rad  ac_frequency=0 Hz  noise_mode=ee.enum.sources.noise.Disabled  PSD=0 A^2/Hz  sample_time=1e-3 s  repeatability=ee.enum.sources.repeatability.NotRepeatable  user_seed=0  auto_seed=676943032  i_specify=off  i_priority=None  i=0 A  i_nominal_specify=off  i_nominal_unit=A  i_nominal_value=1  v_specify=off  v_priority=None  v=0 V  v_nominal_specify=off  v_nominal_unit=V  v_nominal_value=1
  Demand : ee_lib/Passive/Inductor  l=L_r H  enable_L_tol=0  L_tol=20  tol_distribution=1  nSigma=4  r=0 Ohm  g=0 1/Ohm  enable_operating_limits=0  operating_limit_action=2  max_working_current=1 A  power_rating=1 W  enable_faults=ee.enum.enable.no  fault_action=simscape.enum.assert.action.none  lambdaPercent=50  k_faulted=0.9999  turnsShort=0  openCct=0  groundShort=0  groundShortG=0 1/Ohm  tau_fault=1e-3 s  fault_trigger=ee.enum.faults.faultTrigger.temporal  t_fault=1 s  max_permissible_voltage=100 V  n_fail_on_voltage=1  max_permissible_current=1 A  t_fail_on_current=1 s  i_L_specify=off  i_L_priority=High  i_L=0 A  i_L_nominal_specify=off  i_L_nominal_unit=A  i_L_nominal_value=1
  Integrator : Integrator
  PS-Simulink Converter : nesl_utility/PS-Simulink Converter  PhysicalDomain=network_engine_domain  SubClassName=ps_output  LeftPortType=input  RightPortType=output  PseudoPeriodic=off  Frequencies=[]  VectorFormat=inherit  Unit=inherit  AffineConversion=off
  PS-Simulink Converter1 : nesl_utility/PS-Simulink Converter  PhysicalDomain=network_engine_domain  SubClassName=ps_output  LeftPortType=input  RightPortType=output  PseudoPeriodic=off  Frequencies=[]  VectorFormat=inherit  Unit=inherit  AffineConversion=off
  PS-Simulink Converter2 : nesl_utility/PS-Simulink Converter  PhysicalDomain=network_engine_domain  SubClassName=ps_output  LeftPortType=input  RightPortType=output  PseudoPeriodic=off  Frequencies=[]  VectorFormat=inherit  Unit=inherit  AffineConversion=off
  "Price " : Scope
  Price dyn : Scope
  Rdam : Scope
  Scope : Scope
  Storage : fl_lib/Electrical/Electrical Elements/Capacitor  c=C_r F  r=0 Ohm  g=0 1/Ohm  i_specify=off  i_priority=None  i=0 A  i_nominal_specify=off  i_nominal_unit=A  i_nominal_value=1  v_specify=off  v_priority=None  v=0 V  v_nominal_specify=off  v_nominal_unit=V  v_nominal_value=1  vc_specify=off  vc_priority=High  vc=0 V  vc_nominal_specify=off  vc_nominal_unit=V  vc_nominal_value=1
  Voltage Sensor1 : fl_lib/Electrical/Electrical Sensors/Voltage Sensor
  "i+ " : PMIOPort  Tag=PMCPort  Side=Left
  i- : PMIOPort  Tag=PMCPort  Port=2  Side=Left
  Out1 : Outport
  Out2 : Outport  Port=2
  wires:
  Integrator/1 -> Out1/1, "Price "/1
  PS-Simulink Converter/1 -> Scope/1
  PS-Simulink Converter2/1 -> Integrator/1, Price dyn/1
  PS-Simulink Converter1/1 -> Out2/1, Rdam/1
  connections:
  Demand/LConn1 -- Current Source/LConn1 -- i-/RConn1 -- Storage/LConn1 -- Voltage Sensor1/LConn1
  Current Sensor/LConn1 -- Voltage Sensor1/RConn2 -- Current Source/RConn1 -- Demand/RConn1 -- Current Sensor1/RConn2
  Storage/RConn1 -- Current Sensor/RConn2
  Voltage Sensor1/RConn1 -- PS-Simulink Converter2/LConn1
  PS-Simulink Converter/LConn1 -- Current Sensor/RConn1
  Current Sensor1/RConn1 -- PS-Simulink Converter1/LConn1
  Current Sensor1/LConn1 -- "i+ "/RConn1

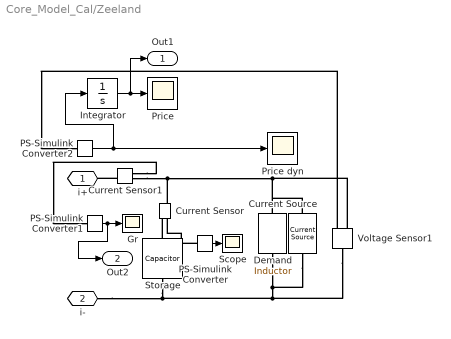
== system Core_Model_Cal/Zeeland ==
  Current Sensor : fl_lib/Electrical/Electrical Sensors/Current Sensor
  Current Sensor1 : fl_lib/Electrical/Electrical Sensors/Current Sensor
  Current Source : ee_lib/Sources/Current Source  dc_current=id_z A  ac_current=0 A  ac_shift=0 rad  ac_frequency=0 Hz  noise_mode=ee.enum.sources.noise.Disabled  PSD=0 A^2/Hz  sample_time=1e-3 s  repeatability=ee.enum.sources.repeatability.NotRepeatable  user_seed=0  auto_seed=4168664255  i_specify=off  i_priority=None  i=0 A  i_nominal_specify=off  i_nominal_unit=A  i_nominal_value=1  v_specify=off  v_priority=None  v=0 V  v_nominal_specify=off  v_nominal_unit=V  v_nominal_value=1
  Demand : ee_lib/Passive/Inductor  l=L_z H  enable_L_tol=0  L_tol=20  tol_distribution=1  nSigma=4  r=0 Ohm  g=0 1/Ohm  enable_operating_limits=0  operating_limit_action=2  max_working_current=1 A  power_rating=1 W  enable_faults=ee.enum.enable.no  fault_action=simscape.enum.assert.action.none  lambdaPercent=50  k_faulted=0.9999  turnsShort=0  openCct=0  groundShort=0  groundShortG=0 1/Ohm  tau_fault=1e-3 s  fault_trigger=ee.enum.faults.faultTrigger.temporal  t_fault=1 s  max_permissible_voltage=100 V  n_fail_on_voltage=1  max_permissible_current=1 A  t_fail_on_current=1 s  i_L_specify=off  i_L_priority=High  i_L=0 A  i_L_nominal_specify=off  i_L_nominal_unit=A  i_L_nominal_value=1
  Gr : Scope
  Integrator : Integrator
  PS-Simulink Converter : nesl_utility/PS-Simulink Converter  PhysicalDomain=network_engine_domain  SubClassName=ps_output  LeftPortType=input  RightPortType=output  PseudoPeriodic=off  Frequencies=[]  VectorFormat=inherit  Unit=inherit  AffineConversion=off
  PS-Simulink Converter1 : nesl_utility/PS-Simulink Converter  PhysicalDomain=network_engine_domain  SubClassName=ps_output  LeftPortType=input  RightPortType=output  PseudoPeriodic=off  Frequencies=[]  VectorFormat=inherit  Unit=inherit  AffineConversion=off
  PS-Simulink Converter2 : nesl_utility/PS-Simulink Converter  PhysicalDomain=network_engine_domain  SubClassName=ps_output  LeftPortType=input  RightPortType=output  PseudoPeriodic=off  Frequencies=[]  VectorFormat=inherit  Unit=inherit  AffineConversion=off
  "Price " : Scope
  Price dyn : Scope
  Scope : Scope
  Storage : fl_lib/Electrical/Electrical Elements/Capacitor  c=C_z F  r=0 Ohm  g=0 1/Ohm  i_specify=off  i_priority=None  i=0 A  i_nominal_specify=off  i_nominal_unit=A  i_nominal_value=1  v_specify=off  v_priority=None  v=0 V  v_nominal_specify=off  v_nominal_unit=V  v_nominal_value=1  vc_specify=off  vc_priority=High  vc=0 V  vc_nominal_specify=off  vc_nominal_unit=V  vc_nominal_value=1
  Voltage Sensor1 : fl_lib/Electrical/Electrical Sensors/Voltage Sensor
  "i+ " : PMIOPort  Tag=PMCPort  Side=Left
  i- : PMIOPort  Tag=PMCPort  Port=2  Side=Left
  Out1 : Outport
  Out2 : Outport  Port=2
  wires:
  Integrator/1 -> Out1/1, "Price "/1
  PS-Simulink Converter/1 -> Scope/1
  PS-Simulink Converter2/1 -> Integrator/1, Price dyn/1
  PS-Simulink Converter1/1 -> Out2/1, Gr/1
  connections:
  Demand/LConn1 -- Current Source/LConn1 -- i-/RConn1 -- Storage/LConn1 -- Voltage Sensor1/LConn1
  Current Sensor/LConn1 -- Voltage Sensor1/RConn2 -- Current Source/RConn1 -- Demand/RConn1 -- Current Sensor1/RConn2
  Storage/RConn1 -- Current Sensor/RConn2
  Voltage Sensor1/RConn1 -- PS-Simulink Converter2/LConn1
  PS-Simulink Converter/LConn1 -- Current Sensor/RConn1
  Current Sensor1/RConn1 -- PS-Simulink Converter1/LConn1
  Current Sensor1/LConn1 -- "i+ "/RConn1

== matlab function Core_Model_Cal/Yearly distribution ==
  data: X input; wind_distr output
function wind_distr= fcn(X)

%% Parameters
a0 = 9.564;
a1 = 1.636;
b1 = 0.4314;
a2 = 0.2612;
b2 = 0.2799;
a3 = -0.4869;
b3 = 0.4023;
a4 = -0.141;
b4 = 0.06985;
a5 = 0.1669;
b5 = 0.03972;
w = 0.01721;

% % c0 = 9.839;
% c1 = 0.2685;
% d1 = -0.1482;
% c2 = -0.08017;
% d2 = -0.08146;
% w2 = 6.288;


       aa0 =       10.21  ;
       aa1 =      0.1631 ;
       bb1 =     -0.2515 ;
       aa2 =    -0.05622  ;
       bb2 =    -0.08132  ;
       aa3 =    -0.01446  ;
       bb3 =     0.01009  ;
       ww =      6.545;
%% Generate wind distributions
yearly_w = a0 + a1*cos(X*w) + b1*sin(X*w) + a2*cos(2*X*w) + b2*sin(2*X*w) + a3*cos(3*X*w) + b3*sin(3*X*w) + a4*cos(4*X*w) + b4*sin(4*X*w) + a5*cos(5*X*w) + b5*sin(5*X*w);
% daily_w = c1*cos(X*w2) + d1*sin(X*w2) + c2*cos(2*X*w2) + d2*sin(2*X*w2);


% Convert X from days to hours by dividing by 24
X_in_hours = X ;

daily_w =  aa1*cos(X_in_hours*ww) + bb1*sin(X_in_hours*ww) + aa2*cos(2*X_in_hours*ww) + bb2*sin(2*X_in_hours*ww) + aa3*cos(3*X_in_hours*ww) + bb3*sin(3*X_in_hours*ww);
    

% Total wind distribution
wind_distr = yearly_w + daily_w; %TNO: Offshore wind energy deployment in the North Sea by 2030: long-term measurement campaign.EPL, 2016-2020

end

== matlab function Core_Model_Cal/Yearly distribution1 ==
  data: wind_distr input; current output
function current= fcn(wind_distr)
wind=wind_distr;

%% Wind to Electricity

       
    % Power curve
    wind_speeds = [0, 2, 4, 6, 8, 10, 12, 14, 16, 18, 20, 22, 24, 26]; % Wind speed values
    power_output = [0, 0, 0.5, 1, 3.7, 4.7, 6.3, 9.5, 9.5, 9.5, 9.5, 9.5, 0, 0]; % Corresponding power output values  in MWh/h
    %powercurve: https://www.researchgate.net/figure/Power-curve-of-the-Vestas-V164-95-turbine-including-some-technical-data-left-side-and_fig4_351600993

    % Interpolate the power curve
    power_curve = interp1(wind_speeds, power_output, wind, 'linear', 'extrap');  % 'extrap' for extrapolation MW/turbine = MW/9.5MW
    
    % Limit power output to positive values
    power_curve(power_curve < 0) = 0;

    % Apply the power curve to wind speed samples
    electricity_production = power_curve .* wind; %MWh/h

    % Consider turbine availability and capacity if applicable
    availability_factor = 1; % Availability factor
    offshore_wind_capacity = 12e3; % Offshore wind capacity in MW (=12GW)
    nr_turbines=offshore_wind_capacity/9.5;
    % offshore_wind_capacity = 30; % Offshore wind capacity in MW

    % Produced electricity
    electricity_production_MW = electricity_production * availability_factor * nr_turbines; %MWh
    electricity_production_GW = electricity_production_MW*1e-3;

    %% Scaling to integrate within the model 
    % current = 2e7 * electricity_production;
    current = electricity_production_GW/26^2; %GWh/h

    % \ 0.0002*30/10*0.5
end
